simulink model "chap1_11"  (Simulink 5.0)
settings: Solver=ode5  StartTime=0.0  StopTime=1  FixedStep=0.001  RelTol=1e-3

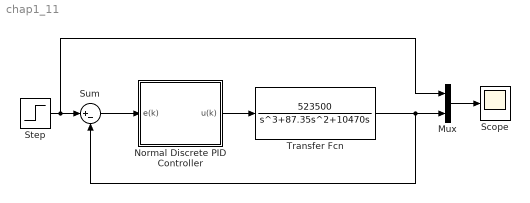
== system chap1_11 ==
  Mux : Mux  Inputs=2
  Normal Discrete PID Controller : Subsystem  AncestorBlock=|  mask{Kp=0.5, Ki=0.001, Kd=0.001, T=0.001, U_m=10}
      | pidblock/Discrete PID
      | Controllers/Normal Discrete
      | PID Controller
      mask prompts: Kp "Proportional Kp"; Ki "Integrator Ki"; Kd "Derivative Kd"; T "Sampling period T"; U_m "Actuator Limit"
      mask Display: disp('Discrete PID')
  Scope : Scope
      settings: TimeRange=1  YMin=-10  YMax=10
  Step : Step  Time=0  SampleTime=0
  Sum : Sum  Inputs=|+-  SaturateOnIntegerOverflow=on
  Transfer Fcn : TransferFcn  Numerator=[523500]  Denominator=[1 87.35 10470 0]
  wires:
  Sum/1 -> Normal Discrete PID Controller/1(e(k))
  Transfer Fcn/1 -> Mux/2, Sum/2
  Step/1 -> Sum/1, Mux/1
  Mux/1 -> Scope/1
  Normal Discrete PID Controller/1(u(k)) -> Transfer Fcn/1

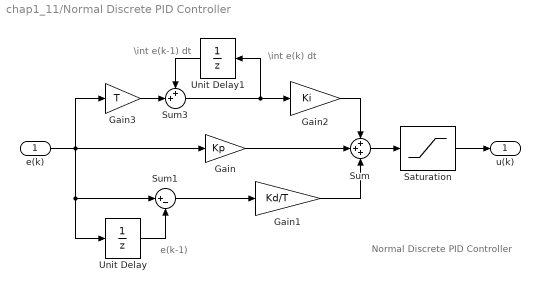
== system chap1_11/Normal Discrete PID Controller ==
  note: \int e(k) dt
  note: Normal Discrete PID Controller
  note: e(k-1)
  note: \int e(k-1) dt
  e(k) : Inport
  Gain : Gain  Gain=Kp  SaturateOnIntegerOverflow=on
  Gain1 : Gain  Gain=Kd/T  SaturateOnIntegerOverflow=on
  Gain2 : Gain  Gain=Ki  SaturateOnIntegerOverflow=on
  Gain3 : Gain  Gain=T  SaturateOnIntegerOverflow=on
  Saturation : Saturate  UpperLimit=U_m  LowerLimit=-U_m
  Sum : Sum  Inputs=+++  SaturateOnIntegerOverflow=on
  Sum1 : Sum  Inputs=|+-  SaturateOnIntegerOverflow=on
  Sum3 : Sum  Inputs=++|  SaturateOnIntegerOverflow=on
  Unit Delay : UnitDelay  SampleTime=-1
  Unit Delay1 : UnitDelay  Orientation=left  SampleTime=-1
  u(k) : Outport
  wires:
  Gain2/1 -> Sum/1
  Sum3/1 -> Gain2/1, Unit Delay1/1
  Unit Delay1/1 -> Sum3/1
  Gain3/1 -> Sum3/2
  Saturation/1 -> u(k)/1
  Sum/1 -> Saturation/1
  e(k)/1 -> Sum1/1, Unit Delay/1, Gain3/1, Gain/1
  Unit Delay/1 -> Sum1/2
  Sum1/1 -> Gain1/1
  Gain/1 -> Sum/2
  Gain1/1 -> Sum/3
